simulink model "SImonPablo1ej5"  (R2018a)
settings: Solver=VariableStepAuto  StartTime=0.0  StopTime=10.0  RelTol=1e-3
settings Model: Creator=pablo.parada.souto  LastModifiedBy=pablo.parada.souto

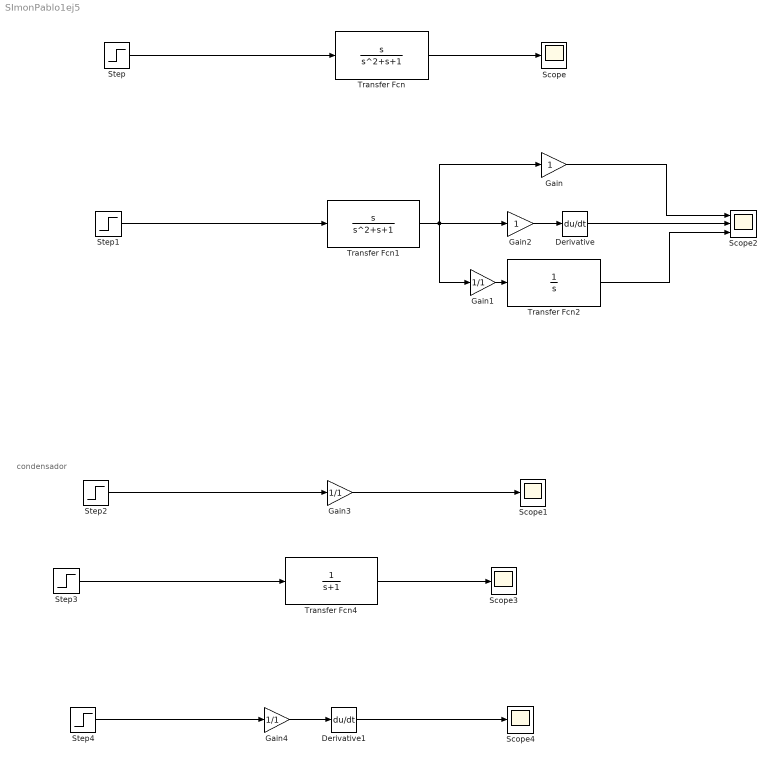
== system SImonPablo1ej5 ==
  note: condensador
  Derivative : Derivative
  Derivative1 : Derivative
  Gain : Gain
  Gain1 : Gain  Gain=1/1
  Gain2 : Gain
  Gain3 : Gain  Gain=1/1
  Gain4 : Gain  Gain=1/1
  Scope{,1,3..4} (4 alike) : Scope
  Scope2 : Scope  NumInputPorts=3
  Step{,1..4} (5 alike) : Step  SampleTime=0
  Transfer Fcn : TransferFcn  Numerator=[1 0]  Denominator=[1 1 1]
  Transfer Fcn1 : TransferFcn  Numerator=[1 0]  Denominator=[1 1 1]
  Transfer Fcn2 : TransferFcn  Numerator=[0 1]  Denominator=[1 0]
  Transfer Fcn4 : TransferFcn  Denominator=[1 1]
  wires:
  Step/1 -> Transfer Fcn/1
  Transfer Fcn/1 -> Scope/1
  Step1/1 -> Transfer Fcn1/1
  Transfer Fcn1/1 -> Gain1/1, Gain2/1, Gain/1
  Derivative/1 -> Scope2/2
  Gain/1 -> Scope2/1
  Transfer Fcn2/1 -> Scope2/3
  Gain2/1 -> Derivative/1
  Gain1/1 -> Transfer Fcn2/1
  Gain3/1 -> Scope1/1
  Step2/1 -> Gain3/1
  Transfer Fcn4/1 -> Scope3/1
  Step3/1 -> Transfer Fcn4/1
  Derivative1/1 -> Scope4/1
  Step4/1 -> Gain4/1
  Gain4/1 -> Derivative1/1
